simulink model "ParallelNew"  (R2021b)
settings: Solver=FixedStepAuto  StartTime=0.0  StopTime=17  FixedStep=0.0001  RelTol=1e-3
InitFcn:
  | ra = 4;
  | jm = 0.0000218;
  | rm = 0.7/100;
  | dsm = 62.892;
  | kt = 0.138;
  | ke = kt;
  | ms = 0.93;
  | hl = 1.5 / 100;
  | Lr = 24.1 / 100;
  | Lcm = hl / 2 + Lr;
  | ml =0.182;
  | mr = 0.085;
  | rl = 20.125 / 1000;
  | Jp =1/3 * mr * Lr^2 + 1/2*ml*rl^2 + ml * Lcm ^ 2;
  | Dp = 0.007;
  | g = 9.82;
StartFcn:
  | ra = 4;
  | jm = 0.0000218;
  | rm = 0.7/100;
  | dsm = 62.892;
  | kt = 0.138;
  | ke = kt;
  | ms = 0.93;
undefined symbols (not defined in the file): direction_sign, distance, Dsm, mj, PKd, PKi, PKp, Ra, SKd, SKi, SKp, tau
settings Model: Creator=labadmin  LastModifiedBy=Norbert
settings SolverCC: AlgebraicLoopSolver=TrustRegion
settings DataIOCC: ReturnWorkspaceOutputs=off
settings DebuggingCC: SFMachineParentedDataDiag=warning  ArithmeticOperatorsInVariantConditions=warning
settings SFSimCC: SimUseLocalCustomCode=off  CustomCodeUndefinedFunction=UseInterfaceOnly
settings RTWCC: Description=Simulink Desktop Real-Time  SystemTargetFile=sldrt.tlc  TemplateMakefile=sldrt.tmf  RTWUseLocalCustomCode=off  RTWCompilerOptimization=on
settings CodeAppCC: MaxIdLength=95
settings SimulinkDesktopRealTimeCC: TargetPreCompLibLocation=C:\Program Files\MATLAB\R2021b\toolbox\sldrt\lib\win64

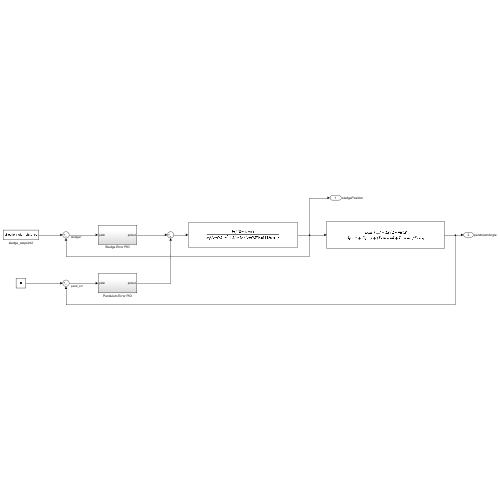
[thumbnail: Simulink's stored preview of the top-level diagram]
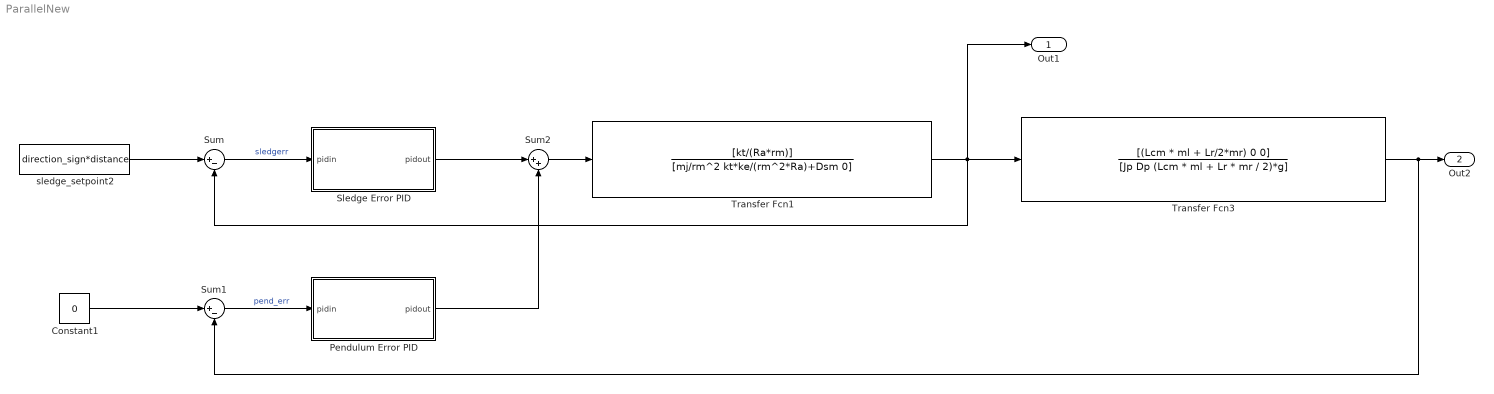
== system ParallelNew ==
  Constant1 : Constant  Value=0
  Pendulum Error PID : Subsystem
  Sledge Error PID : Subsystem
  Sum : Sum  Inputs=|+-
  Sum1 : Sum  Inputs=|+-
  Sum2 : Sum  Inputs=|++
  Transfer Fcn1 : TransferFcn  Numerator=[kt/(Ra*rm)]  Denominator=[mj/rm^2 kt*ke/(rm^2*Ra)+Dsm 0]
  Transfer Fcn3 : TransferFcn  Numerator=[(Lcm * ml + Lr/2*mr) 0 0]  Denominator=[Jp Dp (Lcm * ml + Lr * mr / 2)*g]
  sledge_setpoint2 : Constant  Value=direction_sign*distance
  Out1 : Outport  SignalName=sledgePosition
  Out2 : Outport  Port=2  SignalName=pendulumAngle
  wires:
  sledge_setpoint2/1 -> Sum/1
  Pendulum Error PID/1(pidout) -> Sum2/2
  Sum2/1 -> Transfer Fcn1/1
  Constant1/1 -> Sum1/1
  Sum/1 -> Sledge Error PID/1(pidin)  "sledgerr"
  Sum1/1 -> Pendulum Error PID/1(pidin)  "pend_err"
  Sledge Error PID/1(pidout) -> Sum2/1
  Transfer Fcn1/1 -> Out1/1, Sum/2, Transfer Fcn3/1
  Transfer Fcn3/1 -> Out2/1, Sum1/2

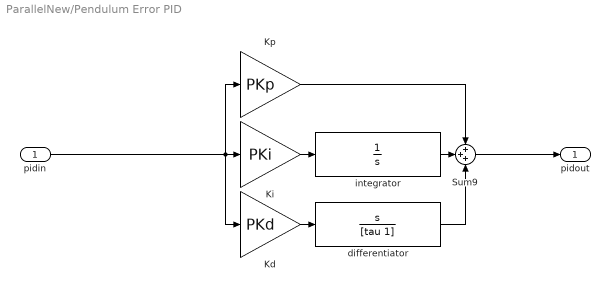
== system ParallelNew/Pendulum Error PID ==
  pidin : Inport
  Kd : Gain  Gain=PKd
  Ki : Gain  Gain=PKi
  Kp : Gain  Gain=PKp
  Sum9 : Sum  Inputs=+++
  differentiator : TransferFcn  Numerator=[1 0]  Denominator=[tau 1]
  integrator : TransferFcn  Denominator=[1 0]
  pidout : Outport  VectorParamsAs1DForOutWhenUnconnected=off
  wires:
  pidin/1 -> Kp/1, Kd/1, Ki/1
  Sum9/1 -> pidout/1
  Kd/1 -> differentiator/1
  Ki/1 -> integrator/1
  Kp/1 -> Sum9/1
  integrator/1 -> Sum9/2
  differentiator/1 -> Sum9/3

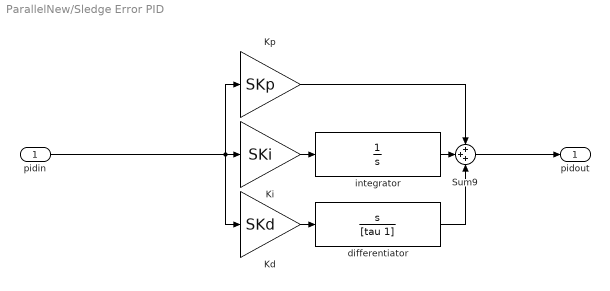
== system ParallelNew/Sledge Error PID ==
  pidin : Inport
  Kd : Gain  Gain=SKd
  Ki : Gain  Gain=SKi
  Kp : Gain  Gain=SKp
  Sum9 : Sum  Inputs=+++
  differentiator : TransferFcn  Numerator=[1 0]  Denominator=[tau 1]
  integrator : TransferFcn  Denominator=[1 0]
  pidout : Outport  VectorParamsAs1DForOutWhenUnconnected=off
  wires:
  pidin/1 -> Kp/1, Kd/1, Ki/1
  Sum9/1 -> pidout/1
  Kd/1 -> differentiator/1
  Ki/1 -> integrator/1
  Kp/1 -> Sum9/1
  integrator/1 -> Sum9/2
  differentiator/1 -> Sum9/3
